simulink model "Tactical_WT_3_15_trainlm_Dec_22"  (R2021a)
settings: Solver=FixedStepAuto  StartTime=0  StopTime=T  FixedStep=Ts  RelTol=1e-3  EnableMultiTasking=on
libraries: neural x50
(part 2 of 2)

== system Tactical_WT_3_15_trainlm_Dec_22/Feed-Forward Neural Network/Layer 3/Delays 1 ==
  "p{3}" : Inport  PortDimensions=15
      mask Display: e = 0.06;c1 = [120 230 180]/255;c2 = ([120 230 180]+0)/(256+128);c3 = ([120 230 180]+128)/(256+128);patch([0 1 1 0],[0 0 1 1],c1);patch([0 1 1 1-e 1-e 0+e],[0 0 1 1-e 0+e 0+e],c2);patch([0 0 1 1-e 0+e 0+e],[0 1 1 1-e 1-e 0+e],c3);plot([0 1 1 0 0],[0 0 1 1 0]);
  mux : Mux  Inputs=1
      mask Display: e = 0.06;c1 = [120 150 230]/255;c2 = ([120 150 230]+0)/383;c3 = ([120 150 230]+128)/383;patch([0 1 1 0],[0 0 1 1],c1);patch([0 1 1 1-e 1-e 0+e],[0 0 1 1-e 0+e 0+e],c2);patch([0 0 1 1-e 0+e 0+e],[0 1 1 1-e 1-e 0+e],c3);plot([0 1 1 0 0],[0 0 1 1 0]);disp('Mux')
  "pd{3,2}" : Outport
      mask Display: e = 0.06;c1 = [120 230 180]/255;c2 = ([120 230 180]+0)/(256+128);c3 = ([120 230 180]+128)/(256+128);patch([0 1 1 0],[0 0 1 1],c1);patch([0 1 1 1-e 1-e 0+e],[0 0 1 1-e 0+e 0+e],c2);patch([0 0 1 1-e 0+e 0+e],[0 1 1 1-e 1-e 0+e],c3);plot([0 1 1 0 0],[0 0 1 1 0]);
  wires:
  "p{3}"/1 -> mux/1
  mux/1 -> "pd{3,2}"/1

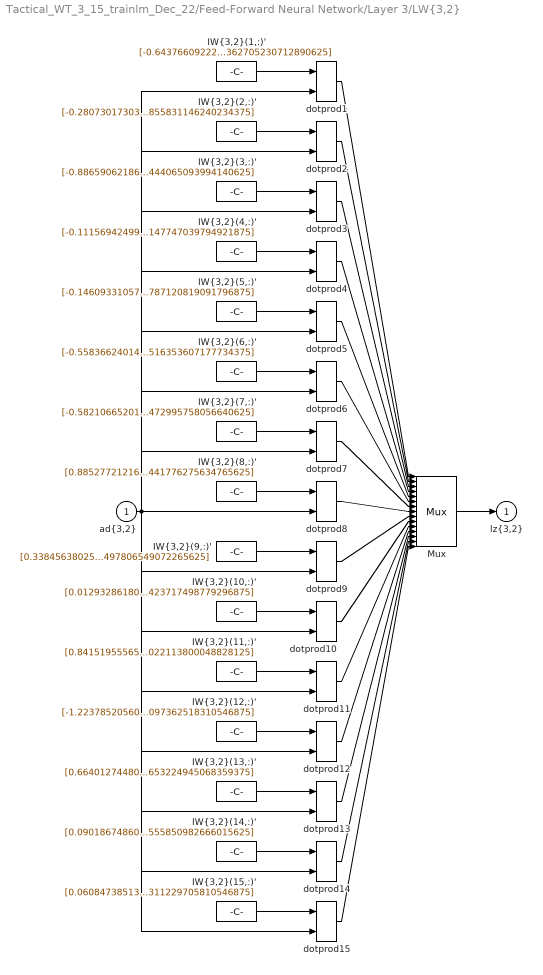
== system Tactical_WT_3_15_trainlm_Dec_22/Feed-Forward Neural Network/Layer 3/LW{3,2} ==
  "ad{3,2}" : Inport  PortDimensions=15
      mask Display: e = 0.06;c1 = [120 230 180]/255;c2 = ([120 230 180]+0)/(256+128);c3 = ([120 230 180]+128)/(256+128);patch([0 1 1 0],[0 0 1 1],c1);patch([0 1 1 1-e 1-e 0+e],[0 0 1 1-e 0+e 0+e],c2);patch([0 0 1 1-e 0+e 0+e],[0 1 1 1-e 1-e 0+e],c3);plot([0 1 1 0 0],[0 0 1 1 0]);
  "IW{3,2}(1,:)'" : Constant  Value=[-0.643766092226467190329231016221456229686737060546875;-0.63161180496894697711240951321087777614593505859375;-0.0878846663125170124430951545946300029754638671875;0.0675439035340004156893201070488430559635162353515625;0.3850639727730376105085952076478861272335052490234375;-0.897336227775257899708094555535353720188140869140625;0.4800646559755552544856982422061264514923095703125;-0.5886509570704803184781894742627628147602081298828125;-0.7754320756879466980393544872640632092952728271484375;-0.0247924491321527273868241536547429859638214111328125;-0.81529532256159686909313677460886538028717041015625;-0.367142001707418064171406513196416199207305908203125;0.9758694699049907939070180873386561870574951171875;-0.2984465102282147785928145822254009544849395751953125;-0.750254482560374302835271009826101362705230712890625]
      mask Display: e = 0.06;c1 = [120 150 230]/255;c2 = ([120 150 230]+0)/383;c3 = ([120 150 230]+128)/383;patch([0 1 1 0],[0 0 1 1],c1);patch([0 1 1 1-e 1-e 0+e],[0 0 1 1-e 0+e 0+e],c2);patch([0 0 1 1-e 0+e 0+e],[0 1 1 1-e 1-e 0+e],c3);plot([0 1 1 0 0],[0 0 1 1 0]);disp('weights');
  "IW{3,2}(10,:)'" : Constant  Value=[0.012932861806001248738962061679558246396481990814208984375;-0.062128653138288573998249120222681085579097270965576171875;0.8771722621157922450407795622595585882663726806640625;-0.455594952849413259432509448743076063692569732666015625;-0.350902559901917709961338687207899056375026702880859375;-0.84536186550799474748174588967231102287769317626953125;-0.6463162781831275349730958623695187270641326904296875;-0.342630248692202321603161863095010630786418914794921875;0.3490652874726027921070681259152479469776153564453125;-0.62823951263718214033104914051364175975322723388671875;-1.1386492687231843934370090209995396435260772705078125;1.1650918873339815018397302992525510489940643310546875;0.758127658513895852365749306045472621917724609375;-0.00796975962872221478650036630142494686879217624664306640625;0.07907052722778488973442989617979037575423717498779296875]
      mask Display: e = 0.06;c1 = [120 150 230]/255;c2 = ([120 150 230]+0)/383;c3 = ([120 150 230]+128)/383;patch([0 1 1 0],[0 0 1 1],c1);patch([0 1 1 1-e 1-e 0+e],[0 0 1 1-e 0+e 0+e],c2);patch([0 0 1 1-e 0+e 0+e],[0 1 1 1-e 1-e 0+e],c3);plot([0 1 1 0 0],[0 0 1 1 0]);disp('weights');
  "IW{3,2}(11,:)'" : Constant  Value=[0.84151955565504155121203666567453183233737945556640625;-1.0663035976051025155442175673670135438442230224609375;0.034794264099935155731824210079139447771012783050537109375;0.005074077723739246238709998948479551472701132297515869140625;-0.170583577201507186060780441039241850376129150390625;0.46417939640432537284908676156192086637020111083984375;0.5787278872838108600973328066174872219562530517578125;-0.5252539605888415508161415345966815948486328125;-0.576942914334483969440725559252314269542694091796875;-0.384747616614892262720815097054583020508289337158203125;-0.67535663681918667311521176088717766106128692626953125;0.59424413476860615812569221816374920308589935302734375;-0.65286617938471891431362337243626825511455535888671875;-0.375132579103413299481672993351821787655353546142578125;0.294427775520772982975614695533295162022113800048828125]
      mask Display: e = 0.06;c1 = [120 150 230]/255;c2 = ([120 150 230]+0)/383;c3 = ([120 150 230]+128)/383;patch([0 1 1 0],[0 0 1 1],c1);patch([0 1 1 1-e 1-e 0+e],[0 0 1 1-e 0+e 0+e],c2);patch([0 0 1 1-e 0+e 0+e],[0 1 1 1-e 1-e 0+e],c3);plot([0 1 1 0 0],[0 0 1 1 0]);disp('weights');
  "IW{3,2}(12,:)'" : Constant  Value=[-1.2237852056045495086067376178107224404811859130859375;0.79700146555187789676466536548105068504810333251953125;-0.6481530102746362320687012470443733036518096923828125;1.0015361879978235126742447391734458506107330322265625;-0.0748081145840246708456078295057523064315319061279296875;-0.08741821491704683533274788942435407079756259918212890625;0.00193690924046334964937765565906602205359376966953277587890625;-0.0581756568660796447023386690489132888615131378173828125;1.300118461194928354274225057451985776424407958984375;0.22715580163557458348577711149118840694427490234375;-0.5346747710031143352438220972544513642787933349609375;-0.49040006084727638668852023329236544668674468994140625;-0.041149067015167205274561723626902676187455654144287109375;0.330995604903117912609644690746790729463100433349609375;0.5452996235336040609098517961683683097362518310546875]
      mask Display: e = 0.06;c1 = [120 150 230]/255;c2 = ([120 150 230]+0)/383;c3 = ([120 150 230]+128)/383;patch([0 1 1 0],[0 0 1 1],c1);patch([0 1 1 1-e 1-e 0+e],[0 0 1 1-e 0+e 0+e],c2);patch([0 0 1 1-e 0+e 0+e],[0 1 1 1-e 1-e 0+e],c3);plot([0 1 1 0 0],[0 0 1 1 0]);disp('weights');
  "IW{3,2}(13,:)'" : Constant  Value=[0.66401274480780625442122300228220410645008087158203125;-0.67520287405773082856086375613813288509845733642578125;-1.214351701776323455561623632092960178852081298828125;0.743175232976401201057115031289868056774139404296875;0.7809513583688765248069785229745320975780487060546875;0.438214556462241666690005104101146571338176727294921875;-0.2340527279122629755736539891586289741098880767822265625;-0.81700253732117555927061403053812682628631591796875;-0.80565808191380361424904776868061162531375885009765625;0.417052393819940359076525737691554240882396697998046875;-0.5722315248044116398062897133058868348598480224609375;-0.388902704068824267569226549312588758766651153564453125;-0.6645861656076454959674038036609999835491180419921875;0.49327395078006641693235678758355788886547088623046875;0.454362410692565443781631984165869653224945068359375]
      mask Display: e = 0.06;c1 = [120 150 230]/255;c2 = ([120 150 230]+0)/383;c3 = ([120 150 230]+128)/383;patch([0 1 1 0],[0 0 1 1],c1);patch([0 1 1 1-e 1-e 0+e],[0 0 1 1-e 0+e 0+e],c2);patch([0 0 1 1-e 0+e 0+e],[0 1 1 1-e 1-e 0+e],c3);plot([0 1 1 0 0],[0 0 1 1 0]);disp('weights');
  "IW{3,2}(14,:)'" : Constant  Value=[0.0901867486025959286255471170079545117914676666259765625;-0.6659724431966862479015389908454380929470062255859375;1.60016888669220680441185322706587612628936767578125;0.70174682667117405099332927420618943870067596435546875;0.2761399714094412427556335387635044753551483154296875;0.5316079186365494368970985306077636778354644775390625;-0.74653620705461742890207688105874694883823394775390625;-0.189369160238817446639814079389907419681549072265625;0.00457508120647607575970372550955289625562727451324462890625;-0.960373372811225589629202659125439822673797607421875;-0.4643817616742713649813367737806402146816253662109375;-0.62640077346045031081445131349028088152408599853515625;1.012597170950646496834224308258853852748870849609375;0.192080901137729964656131187439314089715480804443359375;-0.4101048590528846293778997278423048555850982666015625]
      mask Display: e = 0.06;c1 = [120 150 230]/255;c2 = ([120 150 230]+0)/383;c3 = ([120 150 230]+128)/383;patch([0 1 1 0],[0 0 1 1],c1);patch([0 1 1 1-e 1-e 0+e],[0 0 1 1-e 0+e 0+e],c2);patch([0 0 1 1-e 0+e 0+e],[0 1 1 1-e 1-e 0+e],c3);plot([0 1 1 0 0],[0 0 1 1 0]);disp('weights');
  "IW{3,2}(15,:)'" : Constant  Value=[0.0608473851325773973375277137165539897978305816650390625;-0.415339890138117062701184067918802611529827117919921875;0.476594718757643087680975213515921495854854583740234375;-0.6264445617433178625788059434853494167327880859375;0.41579512909942428766640887261019088327884674072265625;0.049198628305614243438892430049236281774938106536865234375;0.373360179976927053502322451095096766948699951171875;-0.69506564365131195959435217446298338472843170166015625;0.5115379301965090608206310207606293261051177978515625;-0.72383045193070671974311380836297757923603057861328125;-0.520603805098987404420540769933722913265228271484375;0.1370597888159094390747583247502916492521762847900390625;0.456229010786050881431918924135970883071422576904296875;-0.372140393301797434144617682250100187957286834716796875;0.323384093572697206564470207013073377311229705810546875]
      mask Display: e = 0.06;c1 = [120 150 230]/255;c2 = ([120 150 230]+0)/383;c3 = ([120 150 230]+128)/383;patch([0 1 1 0],[0 0 1 1],c1);patch([0 1 1 1-e 1-e 0+e],[0 0 1 1-e 0+e 0+e],c2);patch([0 0 1 1-e 0+e 0+e],[0 1 1 1-e 1-e 0+e],c3);plot([0 1 1 0 0],[0 0 1 1 0]);disp('weights');
  "IW{3,2}(2,:)'" : Constant  Value=[-0.2807301730358393587749787911889143288135528564453125;0.19442270067570976976867314078845083713531494140625;-0.7966612127504897333807321047061122953891754150390625;-0.7816915759150828701962154809734784066677093505859375;0.1133396699280251329611246546846814453601837158203125;-0.854229401802047760838831891305744647979736328125;-0.530346170504191416483763532596640288829803466796875;-0.2234567379043965740237354111741296947002410888671875;0.5688557814878254514923128226655535399913787841796875;0.5379165281177382684774102017399854958057403564453125;-0.9843594128613302185470956828794442117214202880859375;-0.564873381154358700229067835607565939426422119140625;-0.6591359538862333611319854753674007952213287353515625;0.3710714174950744403957969552720896899700164794921875;-0.951131967899252028786349910660646855831146240234375]
      mask Display: e = 0.06;c1 = [120 150 230]/255;c2 = ([120 150 230]+0)/383;c3 = ([120 150 230]+128)/383;patch([0 1 1 0],[0 0 1 1],c1);patch([0 1 1 1-e 1-e 0+e],[0 0 1 1-e 0+e 0+e],c2);patch([0 0 1 1-e 0+e 0+e],[0 1 1 1-e 1-e 0+e],c3);plot([0 1 1 0 0],[0 0 1 1 0]);disp('weights');
  "IW{3,2}(3,:)'" : Constant  Value=[-0.8865906218634176383375233854167163372039794921875;-0.413261978852091205194341227979748509824275970458984375;0.94456433005765216837090747503680177032947540283203125;0.64293239677309899082757738142390735447406768798828125;-0.20695841483681487460444259340874850749969482421875;-0.797085113431229341784955977345816791057586669921875;0.4699150833921044156937796287820674479007720947265625;0.103557063914454960951161410775966942310333251953125;-0.30024237805414732971343028111732564866542816162109375;-0.2079865095642496886085837104474194347858428955078125;-0.1537812296716669635543439653702080249786376953125;-0.5057203121049973493228435472701676189899444580078125;-0.50360032498479101459309958954690955579280853271484375;-0.4117027324643007801796557032503187656402587890625;-0.4196294697385456462512820507981814444065093994140625]
      mask Display: e = 0.06;c1 = [120 150 230]/255;c2 = ([120 150 230]+0)/383;c3 = ([120 150 230]+128)/383;patch([0 1 1 0],[0 0 1 1],c1);patch([0 1 1 1-e 1-e 0+e],[0 0 1 1-e 0+e 0+e],c2);patch([0 0 1 1-e 0+e 0+e],[0 1 1 1-e 1-e 0+e],c3);plot([0 1 1 0 0],[0 0 1 1 0]);disp('weights');
  "IW{3,2}(4,:)'" : Constant  Value=[-0.111569424993383570221539002886856906116008758544921875;-0.75498538634040723849238929687999188899993896484375;-0.543462049102758637530996566056273877620697021484375;-0.210692384652975850389822198849287815392017364501953125;-0.9855000773242801326290418728603981435298919677734375;0.6744866219862479805868815674330107867717742919921875;0.8671119598547323281678700368502177298069000244140625;-0.54918245823905975644407817526371218264102935791015625;0.40460447295680268542383828389574773609638214111328125;-0.44576542761330861797119951006607152521610260009765625;0.2347558951717003683512530187726952135562896728515625;0.52538060943801700997113357516354881227016448974609375;-0.1831188456138839459885758742530015297234058380126953125;-0.09075224905708413614124907553559751249849796295166015625;-0.32993489476157555895241557664121501147747039794921875]
      mask Display: e = 0.06;c1 = [120 150 230]/255;c2 = ([120 150 230]+0)/383;c3 = ([120 150 230]+128)/383;patch([0 1 1 0],[0 0 1 1],c1);patch([0 1 1 1-e 1-e 0+e],[0 0 1 1-e 0+e 0+e],c2);patch([0 0 1 1-e 0+e 0+e],[0 1 1 1-e 1-e 0+e],c3);plot([0 1 1 0 0],[0 0 1 1 0]);disp('weights');
  "IW{3,2}(5,:)'" : Constant  Value=[-0.146093310579803292714728968348936177790164947509765625;-0.359361339256983158829683588919579051434993743896484375;-0.378462785343928576065053448473918251693248748779296875;-0.34436482569002091480570015846751630306243896484375;0.77389233913469401837659233933663927018642425537109375;1.142809078673357792155229617492295801639556884765625;0.6367529423049573811255186228663660585880279541015625;0.33317853426014598650084508335567079484462738037109375;0.8139703312286250547202826055581681430339813232421875;-0.6881763598108960877652862109243869781494140625;0.37069282832645555902928435898502357304096221923828125;0.972553902596783093059684688341803848743438720703125;-0.445743374358037069971061328033101744949817657470703125;1.0341120873192541917973130694008432328701019287109375;0.0229643090386150265647113855038696783594787120819091796875]
      mask Display: e = 0.06;c1 = [120 150 230]/255;c2 = ([120 150 230]+0)/383;c3 = ([120 150 230]+128)/383;patch([0 1 1 0],[0 0 1 1],c1);patch([0 1 1 1-e 1-e 0+e],[0 0 1 1-e 0+e 0+e],c2);patch([0 0 1 1-e 0+e 0+e],[0 1 1 1-e 1-e 0+e],c3);plot([0 1 1 0 0],[0 0 1 1 0]);disp('weights');
  "IW{3,2}(6,:)'" : Constant  Value=[-0.5583662401458315827085243654437363147735595703125;0.7124365525745333105334111678530462086200714111328125;-0.96199448481999849658308221478364430367946624755859375;0.10709633240120673691730956988976686261594295501708984375;-0.331167533680728765066447749632061459124088287353515625;0.4052850639894625128789584778132848441600799560546875;-1.020250542652671565946320697548799216747283935546875;-0.0893490960573140868827834992771386168897151947021484375;-0.1502061968489028787043793045086204074323177337646484375;0.478076440819727832565178005097550339996814727783203125;0.26430534985612175180591520984307862818241119384765625;0.460568940625738443284120648968382738530635833740234375;0.49507474578665144893108163159922696650028228759765625;0.58248125018344676373516222156467847526073455810546875;0.795041702775785008583397939219139516353607177734375]
      mask Display: e = 0.06;c1 = [120 150 230]/255;c2 = ([120 150 230]+0)/383;c3 = ([120 150 230]+128)/383;patch([0 1 1 0],[0 0 1 1],c1);patch([0 1 1 1-e 1-e 0+e],[0 0 1 1-e 0+e 0+e],c2);patch([0 0 1 1-e 0+e 0+e],[0 1 1 1-e 1-e 0+e],c3);plot([0 1 1 0 0],[0 0 1 1 0]);disp('weights');
  "IW{3,2}(7,:)'" : Constant  Value=[-0.582106652013729242156614418490789830684661865234375;-0.8570943744259109653427231023670174181461334228515625;-0.40351205622447228194005219847895205020904541015625;-0.979326763313207226957501916331239044666290283203125;0.215731814525891518741218533250503242015838623046875;-0.735834088572874467359952177503146231174468994140625;-0.2671267673616022353400012434576638042926788330078125;-0.6963089497674668226778749158256687223911285400390625;0.3895043892358802661846084447461180388927459716796875;-0.14087108149629390396739836432971060276031494140625;-0.782364123453909154903840317274443805217742919921875;-0.631132664484693517437108312151394784450531005859375;-0.19522333460767615775921512977220118045806884765625;-0.3293773385895077954188536750734783709049224853515625;0.8714617455697608594533676296123303472995758056640625]
      mask Display: e = 0.06;c1 = [120 150 230]/255;c2 = ([120 150 230]+0)/383;c3 = ([120 150 230]+128)/383;patch([0 1 1 0],[0 0 1 1],c1);patch([0 1 1 1-e 1-e 0+e],[0 0 1 1-e 0+e 0+e],c2);patch([0 0 1 1-e 0+e 0+e],[0 1 1 1-e 1-e 0+e],c3);plot([0 1 1 0 0],[0 0 1 1 0]);disp('weights');
  "IW{3,2}(8,:)'" : Constant  Value=[0.88527721216646515500769965001381933689117431640625;-0.42192228965260791806457518759998492896556854248046875;-0.76275909937243724368016728476504795253276824951171875;-0.68319161074741641126450986121199093759059906005859375;0.53172798309509061720490308289299719035625457763671875;0.8062292925963585599191674191388301551342010498046875;-0.258140107643199778753029249855899251997470855712890625;0.5648646073642396014946598370443098247051239013671875;0.1919582997568446691705190687571302987635135650634765625;0.1230007587511048050554762767205829732120037078857421875;0.145138315612892865313909851465723477303981781005859375;0.045423058179949467316749434075973113067448139190673828125;1.5358559512927973944584891796694137156009674072265625;-0.29977683443745195557283977905171923339366912841796875;-0.05763188421005017991749497241471544839441776275634765625]
      mask Display: e = 0.06;c1 = [120 150 230]/255;c2 = ([120 150 230]+0)/383;c3 = ([120 150 230]+128)/383;patch([0 1 1 0],[0 0 1 1],c1);patch([0 1 1 1-e 1-e 0+e],[0 0 1 1-e 0+e 0+e],c2);patch([0 0 1 1-e 0+e 0+e],[0 1 1 1-e 1-e 0+e],c3);plot([0 1 1 0 0],[0 0 1 1 0]);disp('weights');
  "IW{3,2}(9,:)'" : Constant  Value=[0.3384563802503179896774554435978643596172332763671875;-0.88130142446556314350658567491336725652217864990234375;-0.052395300526747880243139121603235253132879734039306640625;0.293660764518320405169760078933904878795146942138671875;-0.7903735160530007686219278184580616652965545654296875;-0.81546265042314158844050098196021281182765960693359375;0.3700569453232185335167514494969509541988372802734375;-0.7987873552751569850016721829888410866260528564453125;-0.058671888373387860726726472648806520737707614898681640625;0.21114946967195347138357419680687598884105682373046875;-0.74103316870439794872282845972222276031970977783203125;-0.8453063837746463971001276149763725697994232177734375;-0.244316490697525090514119483486865647137165069580078125;-0.0948149168613519055526239753817208111286163330078125;-0.51858942500223526028690912426100112497806549072265625]
      mask Display: e = 0.06;c1 = [120 150 230]/255;c2 = ([120 150 230]+0)/383;c3 = ([120 150 230]+128)/383;patch([0 1 1 0],[0 0 1 1],c1);patch([0 1 1 1-e 1-e 0+e],[0 0 1 1-e 0+e 0+e],c2);patch([0 0 1 1-e 0+e 0+e],[0 1 1 1-e 1-e 0+e],c3);plot([0 1 1 0 0],[0 0 1 1 0]);disp('weights');
  Mux : Mux  Inputs=15
      mask Display: e = 0.06;c1 = [120 150 230]/255;c2 = ([120 150 230]+0)/383;c3 = ([120 150 230]+128)/383;patch([0 1 1 0],[0 0 1 1],c1);patch([0 1 1 1-e 1-e 0+e],[0 0 1 1-e 0+e 0+e],c2);patch([0 0 1 1-e 0+e 0+e],[0 1 1 1-e 1-e 0+e],c3);plot([0 1 1 0 0],[0 0 1 1 0]);disp('Mux');
  dotprod{1..15} (15 alike) : neural/Weight Functions/dotprod
  "lz{3,2}" : Outport
      mask Display: e = 0.06;c1 = [120 230 180]/255;c2 = ([120 230 180]+0)/(256+128);c3 = ([120 230 180]+128)/(256+128);patch([0 1 1 0],[0 0 1 1],c1);patch([0 1 1 1-e 1-e 0+e],[0 0 1 1-e 0+e 0+e],c2);patch([0 0 1 1-e 0+e 0+e],[0 1 1 1-e 1-e 0+e],c3);plot([0 1 1 0 0],[0 0 1 1 0]);
  wires:
  "IW{3,2}(1,:)'"/1 -> dotprod1/1
  "ad{3,2}"/1 -> dotprod1/2, dotprod2/2, dotprod3/2, dotprod4/2, dotprod5/2, dotprod6/2, dotprod7/2, dotprod8/2, dotprod9/2, dotprod10/2, dotprod11/2, dotprod12/2, dotprod13/2, dotprod14/2, dotprod15/2
  dotprod1/1 -> Mux/1
  "IW{3,2}(2,:)'"/1 -> dotprod2/1
  dotprod2/1 -> Mux/2
  "IW{3,2}(3,:)'"/1 -> dotprod3/1
  dotprod3/1 -> Mux/3
  "IW{3,2}(4,:)'"/1 -> dotprod4/1
  dotprod4/1 -> Mux/4
  "IW{3,2}(5,:)'"/1 -> dotprod5/1
  dotprod5/1 -> Mux/5
  "IW{3,2}(6,:)'"/1 -> dotprod6/1
  dotprod6/1 -> Mux/6
  "IW{3,2}(7,:)'"/1 -> dotprod7/1
  dotprod7/1 -> Mux/7
  "IW{3,2}(8,:)'"/1 -> dotprod8/1
  dotprod8/1 -> Mux/8
  "IW{3,2}(9,:)'"/1 -> dotprod9/1
  dotprod9/1 -> Mux/9
  "IW{3,2}(10,:)'"/1 -> dotprod10/1
  dotprod10/1 -> Mux/10
  "IW{3,2}(11,:)'"/1 -> dotprod11/1
  dotprod11/1 -> Mux/11
  "IW{3,2}(12,:)'"/1 -> dotprod12/1
  dotprod12/1 -> Mux/12
  "IW{3,2}(13,:)'"/1 -> dotprod13/1
  dotprod13/1 -> Mux/13
  "IW{3,2}(14,:)'"/1 -> dotprod14/1
  dotprod14/1 -> Mux/14
  "IW{3,2}(15,:)'"/1 -> dotprod15/1
  dotprod15/1 -> Mux/15
  Mux/1 -> "lz{3,2}"/1

== system Tactical_WT_3_15_trainlm_Dec_22/Feed-Forward Neural Network/Layer 4/Delays 1 ==
  "p{4}" : Inport  PortDimensions=15
      mask Display: e = 0.06;c1 = [120 230 180]/255;c2 = ([120 230 180]+0)/(256+128);c3 = ([120 230 180]+128)/(256+128);patch([0 1 1 0],[0 0 1 1],c1);patch([0 1 1 1-e 1-e 0+e],[0 0 1 1-e 0+e 0+e],c2);patch([0 0 1 1-e 0+e 0+e],[0 1 1 1-e 1-e 0+e],c3);plot([0 1 1 0 0],[0 0 1 1 0]);
  mux : Mux  Inputs=1
      mask Display: e = 0.06;c1 = [120 150 230]/255;c2 = ([120 150 230]+0)/383;c3 = ([120 150 230]+128)/383;patch([0 1 1 0],[0 0 1 1],c1);patch([0 1 1 1-e 1-e 0+e],[0 0 1 1-e 0+e 0+e],c2);patch([0 0 1 1-e 0+e 0+e],[0 1 1 1-e 1-e 0+e],c3);plot([0 1 1 0 0],[0 0 1 1 0]);disp('Mux')
  "pd{4,3}" : Outport
      mask Display: e = 0.06;c1 = [120 230 180]/255;c2 = ([120 230 180]+0)/(256+128);c3 = ([120 230 180]+128)/(256+128);patch([0 1 1 0],[0 0 1 1],c1);patch([0 1 1 1-e 1-e 0+e],[0 0 1 1-e 0+e 0+e],c2);patch([0 0 1 1-e 0+e 0+e],[0 1 1 1-e 1-e 0+e],c3);plot([0 1 1 0 0],[0 0 1 1 0]);
  wires:
  "p{4}"/1 -> mux/1
  mux/1 -> "pd{4,3}"/1

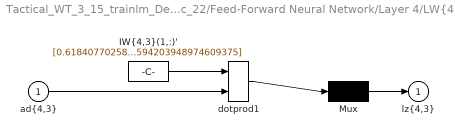
== system Tactical_WT_3_15_trainlm_Dec_22/Feed-Forward Neural Network/Layer 4/LW{4,3} ==
  "ad{4,3}" : Inport  PortDimensions=15
      mask Display: e = 0.06;c1 = [120 230 180]/255;c2 = ([120 230 180]+0)/(256+128);c3 = ([120 230 180]+128)/(256+128);patch([0 1 1 0],[0 0 1 1],c1);patch([0 1 1 1-e 1-e 0+e],[0 0 1 1-e 0+e 0+e],c2);patch([0 0 1 1-e 0+e 0+e],[0 1 1 1-e 1-e 0+e],c3);plot([0 1 1 0 0],[0 0 1 1 0]);
  "IW{4,3}(1,:)'" : Constant  Value=[0.61840770258758670507859278586693108081817626953125;0.4972377435523942512674011595663614571094512939453125;-0.52496017615470036421498889467329718172550201416015625;0.1904621413509307303879580786087899468839168548583984375;-0.316643751206460322134006446503917686641216278076171875;-0.00929272484615830361709409856985075748525559902191162109375;-0.20223849523360204472055556834675371646881103515625;-0.4158839305102379757528296977397985756397247314453125;-0.6249926113958477191800966465962119400501251220703125;-1.2809373657884322028621681965887546539306640625;-0.6491729251225730745744613159331493079662322998046875;0.7914658394398002005942771575064398348331451416015625;1.2034837994186065035506771891959942877292633056640625;0.9398611897363107203773324727080762386322021484375;0.1092062891766899246359656672211713157594203948974609375]
      mask Display: e = 0.06;c1 = [120 150 230]/255;c2 = ([120 150 230]+0)/383;c3 = ([120 150 230]+128)/383;patch([0 1 1 0],[0 0 1 1],c1);patch([0 1 1 1-e 1-e 0+e],[0 0 1 1-e 0+e 0+e],c2);patch([0 0 1 1-e 0+e 0+e],[0 1 1 1-e 1-e 0+e],c3);plot([0 1 1 0 0],[0 0 1 1 0]);disp('weights');
  Mux : Mux  Inputs=1
      mask Display: e = 0.06;c1 = [120 150 230]/255;c2 = ([120 150 230]+0)/383;c3 = ([120 150 230]+128)/383;patch([0 1 1 0],[0 0 1 1],c1);patch([0 1 1 1-e 1-e 0+e],[0 0 1 1-e 0+e 0+e],c2);patch([0 0 1 1-e 0+e 0+e],[0 1 1 1-e 1-e 0+e],c3);plot([0 1 1 0 0],[0 0 1 1 0]);disp('Mux');
  dotprod1 : neural/Weight Functions/dotprod
  "lz{4,3}" : Outport
      mask Display: e = 0.06;c1 = [120 230 180]/255;c2 = ([120 230 180]+0)/(256+128);c3 = ([120 230 180]+128)/(256+128);patch([0 1 1 0],[0 0 1 1],c1);patch([0 1 1 1-e 1-e 0+e],[0 0 1 1-e 0+e 0+e],c2);patch([0 0 1 1-e 0+e 0+e],[0 1 1 1-e 1-e 0+e],c3);plot([0 1 1 0 0],[0 0 1 1 0]);
  wires:
  "IW{4,3}(1,:)'"/1 -> dotprod1/1
  "ad{4,3}"/1 -> dotprod1/2
  dotprod1/1 -> Mux/1
  Mux/1 -> "lz{4,3}"/1
